simulink model "Iris_PID_Gazebo_Excitation_Linear"  (R2022a)
settings: Solver=VariableStepAuto  StartTime=0.0  StopTime=exc_param.sim_time  RelTol=1e-3
values from neighbouring files (symbols this model uses):
  accel_g = param.g    [DeePC_main.m]
  exc_param = evalin('base', 'exc_param')    [DeePC_Optimizer_osqp.m]    (also in DeePC_main.m = generate_excitation_signal(param, rng_seed, Td, Tini))
  K_pitch = param.K_lqr_outer_loop(3,8)    [DeePC_main.m]
  K_roll = param.K_lqr_outer_loop(2,7)    [DeePC_main.m]
  K_yaw = param.K_lqr_outer_loop(4,9)    [DeePC_main.m]
  Ki_xy = 0    [DeePC_main.m]
  Ki_z = 0    [DeePC_main.m]
  Kp_xy = - param.K_lqr_outer_loop(3,1)/param.K_lqr_outer_loop(2,7)    [DeePC_main.m]
  Kp_z = - param.K_lqr_outer_loop(1,3)    [DeePC_main.m]
  Kv_xy = - param.K_lqr_outer_loop(3,4)/param.K_lqr_outer_loop(2,7)    [DeePC_main.m]
  Kv_z = - param.K_lqr_outer_loop(1,6)    [DeePC_main.m]
  mass = param.nrotor_vehicle_mass_for_controller    [DeePC_main.m]
  param = evalin('base', 'param')    [DeePC_Optimizer_osqp.m]    (also in DeePC_main.m = load_crazyflie_parameters(); DeePC_update_uini_yini.m)
undefined symbols (not defined in the file or in its folder): DiscIntNeverNeededParam
libraries: Crazyflie_Library x1
settings Model: Creator=ezzat  LastModifiedBy=simao
settings SolverCC: AlgebraicLoopSolver=LineSearch
settings DataIOCC: ReturnWorkspaceOutputs=off
settings DebuggingCC: UnconnectedInputMsg=warning  UnconnectedOutputMsg=warning  UnconnectedLineMsg=warning  SFMachineParentedDataDiag=warning  ArithmeticOperatorsInVariantConditions=warning
settings SFSimCC: CustomCodeUndefinedFunction=UseInterfaceOnly

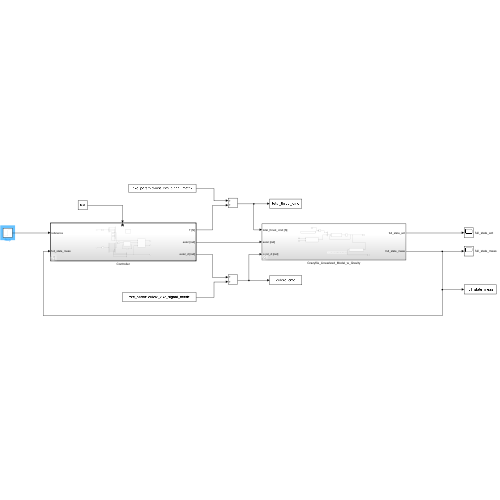
[thumbnail: Simulink's stored preview of the top-level diagram]
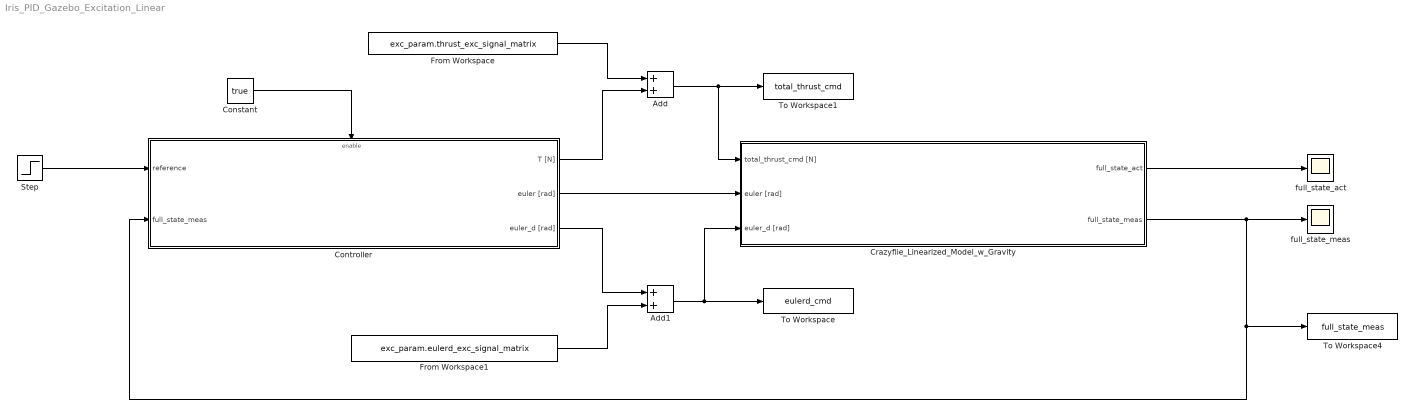
== system Iris_PID_Gazebo_Excitation_Linear ==
  Add : Sum
  Add1 : Sum
  Constant : Constant  Value=true
  Controller : Subsystem  AncestorBlock=Crazyflie_Library/LQR_Controller
  Crazyflie_Linearized_Model_w_Gravity : Subsystem  AncestorBlock=Crazyflie_Library/Crazyflie_Linearized_Model_w_Gravity
  From Workspace : FromWorkspace  VariableName=exc_param.thrust_exc_signal_matrix  SampleTime=exc_param.exc_sample_time  OutputAfterFinalValue=Setting to zero
  From Workspace1 : FromWorkspace  VariableName=exc_param.eulerd_exc_signal_matrix  SampleTime=exc_param.exc_sample_time  OutputAfterFinalValue=Setting to zero
  Step : Step  Time=0  Before=[param.nrotor_initial_condition(1:3); param.nrotor_initial_condition(9)]  After=[param.nrotor_initial_condition(1:3); param.nrotor_initial_condition(9)]  SampleTime=0
  To Workspace : ToWorkspace  VariableName=eulerd_cmd  SampleTime=exc_param.exc_sample_time
  To Workspace1 : ToWorkspace  VariableName=total_thrust_cmd  SampleTime=exc_param.exc_sample_time
  To Workspace4 : ToWorkspace  VariableName=full_state_meas  SampleTime=exc_param.exc_sample_time
  full_state_act : Scope
  full_state_meas : Scope
  wires:
  Crazyflie_Linearized_Model_w_Gravity/1(full_state_act) -> full_state_act/1
  Crazyflie_Linearized_Model_w_Gravity/2(full_state_meas) -> Controller/2(full_state_meas), To Workspace4/1, full_state_meas/1
  Constant/1 -> Controller/Enable
  Step/1 -> Controller/1(reference)
  From Workspace/1 -> Add/1
  From Workspace1/1 -> Add1/2
  Controller/1(T [N]) -> Add/2
  Add/1 -> Crazyflie_Linearized_Model_w_Gravity/1(total_thrust_cmd [N]), To Workspace1/1
  Controller/3(euler_d [rad]) -> Add1/1
  Add1/1 -> To Workspace/1, Crazyflie_Linearized_Model_w_Gravity/3(euler_d [rad])
  Controller/2(euler [rad]) -> Crazyflie_Linearized_Model_w_Gravity/2(euler [rad])

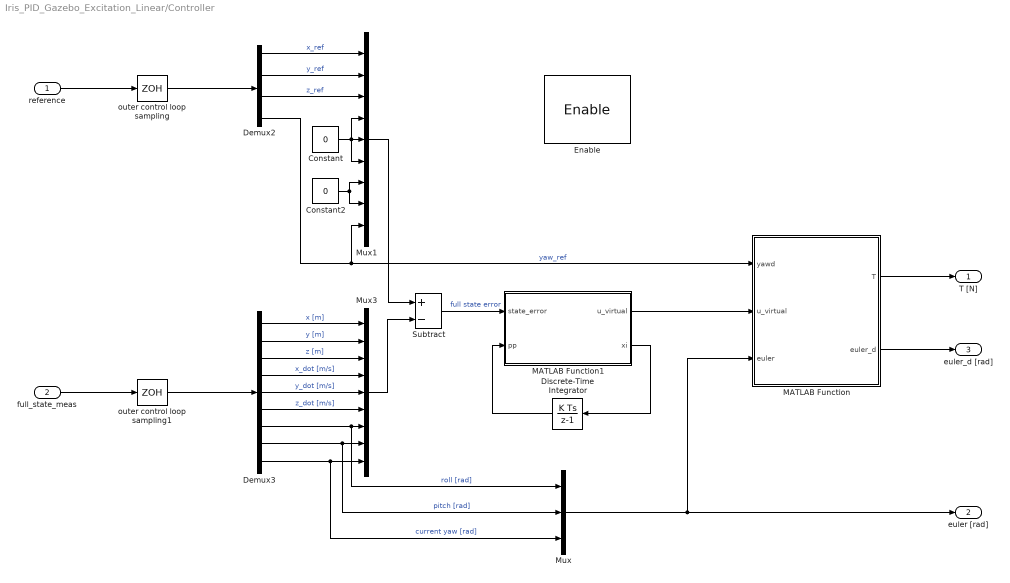
== system Iris_PID_Gazebo_Excitation_Linear/Controller ==
  reference : Inport
  full_state_meas : Inport  Port=2
  Enable : EnablePort
  Constant : Constant  Value=0
  Constant2 : Constant  Value=0
  Demux2 : Demux
  Demux3 : Demux  Outputs=9
  Discrete-Time Integrator : DiscreteIntegrator  InitialCondition=[0;0;0]  SampleTime=-1  ICPrevOutput=DiscIntNeverNeededParam  ICPrevScaledInput=DiscIntNeverNeededParam
  MATLAB Function : MATLAB Function  TreatAsAtomicUnit=on
  MATLAB Function1 : MATLAB Function  TreatAsAtomicUnit=on
  Mux : Mux  Inputs=3
  Mux1 : Mux  Inputs=9
  Mux3 : Mux  Inputs=9
  Subtract : Sum  Inputs=+-
  outer control loop sampling : ZeroOrderHold  SampleTime=param.sample_time_controller_outer
  outer control loop sampling1 : ZeroOrderHold  SampleTime=param.sample_time_controller_outer
  T [N] : Outport
  euler [rad] : Outport  Port=2
  euler_d [rad] : Outport  Port=3
  wires:
  Mux3/1 -> Subtract/2
  Demux2/1 -> Mux1/1  "x_ref"
  Demux3/1 -> Mux3/1  "x [m]"
  Demux3/3 -> Mux3/3  "z [m]"
  Demux3/6 -> Mux3/6  "z_dot [m/s]"
  Constant/1 -> Mux1/5, Mux1/4, Mux1/6
  Constant2/1 -> Mux1/7, Mux1/8
  Demux3/2 -> Mux3/2  "y [m]"
  Demux2/4 -> Mux1/9, MATLAB Function/1(yawd)  "yaw_ref"
  Demux3/8 -> Mux/2, Mux3/8  "pitch [rad]"
  Demux3/9 -> Mux/3, Mux3/9  "current yaw [rad]"
  Demux3/7 -> Mux/1, Mux3/7  "roll [rad]"
  Demux2/2 -> Mux1/2  "y_ref"
  Demux3/4 -> Mux3/4  "x_dot [m/s]"
  Demux2/3 -> Mux1/3  "z_ref"
  Mux1/1 -> Subtract/1
  Demux3/5 -> Mux3/5  "y_dot [m/s]"
  full_state_meas/1 -> outer control loop sampling1/1
  outer control loop sampling/1 -> Demux2/1
  reference/1 -> outer control loop sampling/1
  outer control loop sampling1/1 -> Demux3/1
  Subtract/1 -> MATLAB Function1/1(state_error)  "full state error"
  Mux/1 -> MATLAB Function/3(euler), euler [rad]/1
  MATLAB Function1/2(xi) -> Discrete-Time Integrator/1
  Discrete-Time Integrator/1 -> MATLAB Function1/2(pp)
  MATLAB Function1/1(u_virtual) -> MATLAB Function/2(u_virtual)
  MATLAB Function/1(T) -> T [N]/1
  MATLAB Function/2(euler_d) -> euler_d [rad]/1

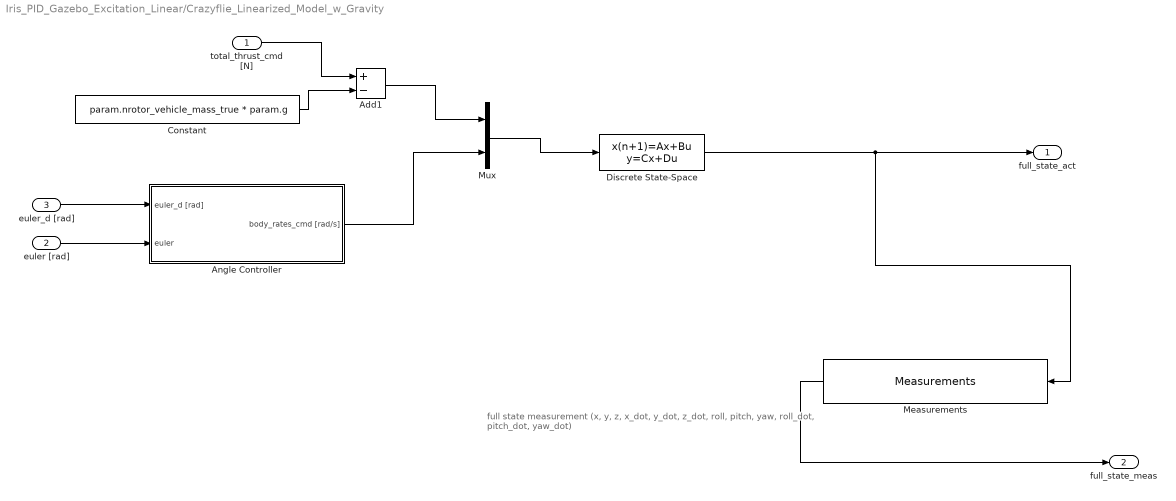
== system Iris_PID_Gazebo_Excitation_Linear/Crazyflie_Linearized_Model_w_Gravity ==
  note: full state measurement
      | (x, y, z, x_dot, y_dot, z_dot, roll, pitch, yaw, roll_dot, pitch_dot, yaw_dot)
  total_thrust_cmd [N] : Inport
  euler [rad] : Inport  Port=2
  euler_d [rad] : Inport  Port=3
  Add1 : Sum  Inputs=+-
  Angle Controller : Subsystem
  Constant : Constant  Value=param.nrotor_vehicle_mass_true * param.g
  Discrete State-Space : DiscreteStateSpace  A=param.Ad_sys  B=param.Bd_sys  C=eye(9)  D=zeros(9,4)  InitialCondition=param.nrotor_initial_condition(1:9)  SampleTime=0.04
  Measurements : Crazyflie_Library/Crazyflie_Linearized_Model_w_Gravity/Measurements  SystemSampleTime=-1  VariantActivationTime=update diagram  Latency=0  AutoFrameSizeCalculation=off
  Mux : Mux  Inputs=2
  full_state_act : Outport  VectorParamsAs1DForOutWhenUnconnected=off
  full_state_meas : Outport  Port=2  VectorParamsAs1DForOutWhenUnconnected=off
  wires:
  Discrete State-Space/1 -> Measurements/1, full_state_act/1
  total_thrust_cmd [N]/1 -> Add1/1
  Add1/1 -> Mux/1
  Constant/1 -> Add1/2
  Mux/1 -> Discrete State-Space/1
  Angle Controller/1(body_rates_cmd [rad/s]) -> Mux/2
  euler_d [rad]/1 -> Angle Controller/1(euler_d [rad])
  euler [rad]/1 -> Angle Controller/2(euler)
  Measurements/1 -> full_state_meas/1

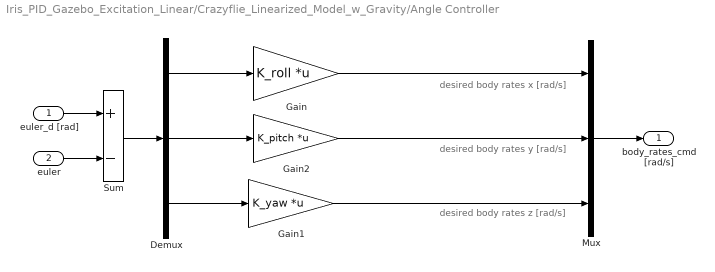
== system Iris_PID_Gazebo_Excitation_Linear/Crazyflie_Linearized_Model_w_Gravity/Angle Controller ==
  note: desired body rates x [rad/s]
  note: desired body rates z [rad/s]
  note: desired body rates y [rad/s]
  euler_d [rad] : Inport
  euler : Inport  Port=2
  Demux : Demux  Outputs=3
  Gain : Gain  Gain=K_roll  Multiplication=Matrix(K*u)
  Gain1 : Gain  Gain=K_yaw  Multiplication=Matrix(K*u)
  Gain2 : Gain  Gain=K_pitch  Multiplication=Matrix(K*u)
  Mux : Mux  Inputs=3
  Sum : Sum  Inputs=+-
  body_rates_cmd [rad/s] : Outport
  wires:
  euler_d [rad]/1 -> Sum/1
  euler/1 -> Sum/2
  Demux/2 -> Gain2/1
  Demux/3 -> Gain1/1
  Mux/1 -> body_rates_cmd [rad/s]/1
  Sum/1 -> Demux/1
  Gain2/1 -> Mux/2
  Gain1/1 -> Mux/3
  Gain/1 -> Mux/1
  Demux/1 -> Gain/1

== matlab function Iris_PID_Gazebo_Excitation_Linear/Controller/MATLAB Function1 ==
  data: state_error input; u_virtual output; pp input; xi output; Kp_xy parameter; Kv_xy parameter; Kp_z parameter; Kv_z parameter; Ki_xy parameter; Ki_z parameter
function [u_virtual,xi] = Controller(state_error, pp, Kp_xy, Kv_xy, Kp_z, Kv_z, Ki_xy, Ki_z)

p_err = state_error(1:3);
v_err = state_error(4:6);

u_virtual = zeros(3,1);
xi = zeros(3,1);

% Kv = -4;
% Kp = -4;
% Ki = 0;
% u = Kp*(p_err) + Kv*(v_err) + Ki*pp;
% u_virtual = u(:);

u_xy = Kv_xy*(v_err(1:2)) + Kp_xy*(p_err(1:2)) + Ki_xy*pp(1:2);

u_z = Kp_z*(p_err(3)) + Kv_z*(v_err(3)) + Ki_z*pp(3);

u_virtual = [u_xy;u_z];

xi = p_err;

== matlab function Iris_PID_Gazebo_Excitation_Linear/Controller/MATLAB Function ==
  data: yawd input; u_virtual input; T output; euler_d output; euler input; mass parameter; accel_g parameter
function [T, euler_d] = input_transform(yawd, u_virtual, euler, mass, accel_g)

T = 0;
euler_d = zeros(3,1);

% Compute pitch, roll and T
Rz = eul2rotm([euler(3,1),0,0],'ZYX');

T_aux = mass * Rz'*(accel_g*[0;0;1] - u_virtual);
% pitchd = atan2(T_aux(1),T_aux(3));
% rolld = atan2(-T_aux(2),norm(T_aux([1,3])));
pitchd = T_aux(1);
rolld = -T_aux(2);

euler_d = [rolld;pitchd;yawd];

% T = norm(T_aux);
T = -u_virtual(3) + mass*accel_g;
